simulink model "Mission_Server_LeaderFollower_QBot2_QDrone_Vicon_FrSky"  (Simulink 9.1)
settings: Solver=ode2  StartTime=0.0  StopTime=inf  FixedStep=0.001  RelTol=1e-3  EnableMultiTasking=on
undefined symbols (not defined in the file): Host, localhost, qc_get_step_size
libraries: quarc_library x34, simulink x5
(part 1 of 2)
settings Model: Creator=Admin  LastModifiedBy=jpineros  SimulationMode=external  ExtModeTrigDuration=10000
settings SolverCC: PositivePriorityOrder=on
settings DataIOCC: SaveFormat=Dataset
settings OptimizationCC: LifeSpan=auto
settings DebuggingCC: UnderspecifiedInitializationDetection=Simplified  MergeDetectMultiDrivingBlocksExec=error
settings HardwareCC: ProdBitPerPointer=64  ProdBitPerSizeT=64  ProdBitPerPtrDiffT=64  ProdLargestAtomicFloat=Float  ProdIntDivRoundTo=Zero  ProdEndianess=LittleEndian  ProdWordSize=64  ProdHWDeviceType=Intel->x86-64 (Windows64)
settings ModelReferenceCC: PropagateSignalLabelsOutOfModel=on
settings RTWCC: SystemTargetFile=quarc_win64.tlc  TemplateMakefile=quarc_default_tmf  Description=QUARC Win64 Target  BuildConfiguration=Faster Runs
settings STFCustomTargetCC: ConcurrentExecutionCompliant=on  SystemTargetFile=quarc_win64.tlc
settings GRTTargetCC: TargetPreCompLibLocation=C:\PROGRA~3\QUARC\lib\2018a\win64\release  ParMdlRefBuildCompliant=off  CompOptLevelCompliant=off  MatFileLogging=off  CPPClassGenCompliant=off  UseToolchainInfoCompliant=off  ExtMode=on  ExtModeMexFile=quarc_comm
settings ConfigComp: CovHtmlReporting=off

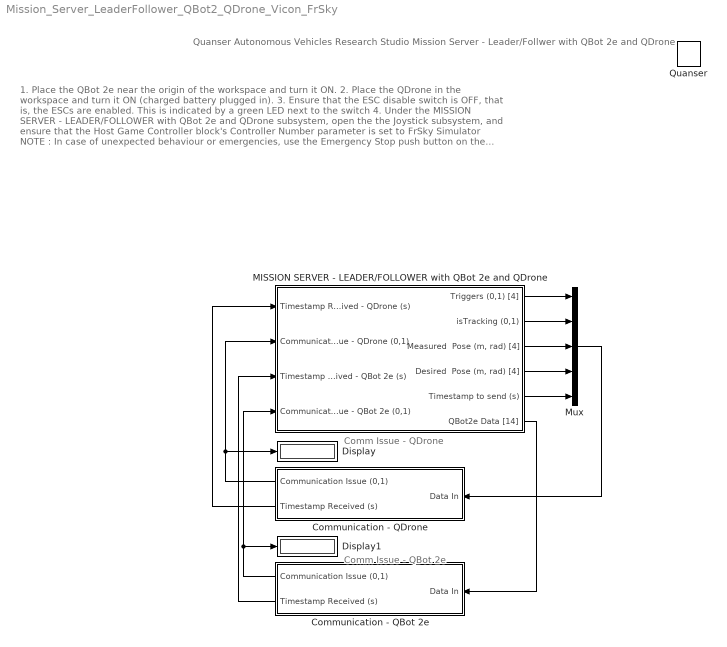
== system Mission_Server_LeaderFollower_QBot2_QDrone_Vicon_FrSky ==
  note: 1. Place the QBot 2e near the origin of the workspace and turn it ON.
      | 2. Place the QDrone in the workspace and turn it ON (charged battery plugged in).
      | 3. Ensure that the ESC disable switch is OFF, that is, the ESCs are enabled. This is indicated by a green LED next to the switch
      | 4. Under the MISSION SERVER - LEADER/FOLLOWER with QBot 2e and QDrone subsystem, open the the Joystick subsystem, and ensure that the Host Game Controller block's Controller Number parameter is set to FrSky Simulator
      | NOTE : In case of unexpected behaviour or emergencies, use the Emergency Stop push button on the Spektrum Joystick to cut all power to the motors (this will result in the drone falling).
      | 5. Open the Data Server (Localization) subsystem and follow the steps there to set up the correct calibration and rigid body definition files for the selected QBot 2e and QDrone.
      | 6. Under the QUARC menu, click on Build .
      | 7. Under the QUARC menu, click on Start . Wait for the model to start running (takes ~1 to 5 seconds for the Motive API to initialize and send localization data).
      | 8. In the MISSION SERVER - LEADER/FOLLOWER with QBot 2e and QDrone subsystem, ensure that the isTracking? display shows 1 and that the Joystick Issue display shows 0 (joystick must be powered ON with USB dongle attached to the PC).
      | 9. Start running the Commander_Stabilizer_QBot2e_Leader.mdl model.
      | 10. Start running the Commander_Stabilizer_QDrone_Follower.mdl model.
      | 11. Arm the drone by moving the Arm/Disarm toggle to the 2 position.
      | 12. Takeoff the drone by moving the Takeoff/Land toggle to the 2 position. The QDrone should takeoff and hover.
      | 13. Toggle the Start/Stop Toggle switch ONCE to start sending waypoint to the Leader (QBot 2e). The QBot 2e should start moving towards the first specified waypoint and the QDrone should follow it.
      | NOTE : The end condition for the FOLLOWER (QDrone) is when the QBot 2e returns to the starting position (when the QDrone model was first started). At that point, the QDrone will be hovering a bit further away (rather than hovering close to/above the QBot 2e) to allow for landing (without hitting the QBot 2e).
      | 14. When finished, move the Takeoff/Land toggle to the 0 position to land the drone. The QDrone should land.
      | 15. Move the Arm/Disarm toggle to the 0 position. (The Commander_Stabilizer_QDrone_Follower.mdl model disarms the drone and stops automatically upon landing).
      | 16. Stop the QBot 2e model. Then stop this model.
  note: Quanser Autonomous Vehicles Research Studio
      | Mission Server - Leader/Follwer with QBot 2e and QDrone
  note: Comm Issue - QDrone
  note: Comm Issue - QBot 2e
  Communication - QBot 2e : Subsystem
  Communication - QDrone : Subsystem
  Display : Display
  Display1 : Display
  MISSION SERVER - LEADER/FOLLOWER with QBot 2e and QDrone : Subsystem
  Mux : Mux  Inputs=5
  Quanser : quarc_library/Logos/Quanser
  wires:
  Communication - QDrone/2(Timestamp Received (s)) -> MISSION SERVER - LEADER/FOLLOWER with QBot 2e and QDrone/1(Timestamp Received - QDrone (s))
  MISSION SERVER - LEADER/FOLLOWER with QBot 2e and QDrone/5(Timestamp to send (s)) -> Mux/5
  Mux/1 -> Communication - QDrone/1(Data In)
  Communication - QDrone/1(Communication Issue (0,1)) -> Display/1, MISSION SERVER - LEADER/FOLLOWER with QBot 2e and QDrone/2(Communication  Issue - QDrone (0,1))
  MISSION SERVER - LEADER/FOLLOWER with QBot 2e and QDrone/3("Measured  Pose (m, rad) [4]") -> Mux/3
  MISSION SERVER - LEADER/FOLLOWER with QBot 2e and QDrone/4("Desired  Pose (m, rad) [4]") -> Mux/4
  Communication - QBot 2e/1(Communication Issue (0,1)) -> MISSION SERVER - LEADER/FOLLOWER with QBot 2e and QDrone/4(Communication  Issue - QBot 2e (0,1)), Display1/1
  Communication - QBot 2e/2(Timestamp Received (s)) -> MISSION SERVER - LEADER/FOLLOWER with QBot 2e and QDrone/3(Timestamp Received - QBot 2e (s))
  MISSION SERVER - LEADER/FOLLOWER with QBot 2e and QDrone/6(QBot2e Data [14]) -> Communication - QBot 2e/1(Data In)
  MISSION SERVER - LEADER/FOLLOWER with QBot 2e and QDrone/1(Triggers (0,1) [4]) -> Mux/1
  MISSION SERVER - LEADER/FOLLOWER with QBot 2e and QDrone/2(isTracking (0,1)) -> Mux/2

== system Mission_Server_LeaderFollower_QBot2_QDrone_Vicon_FrSky/Communication - QBot 2e ==
  note: Argument (-URI_Leader) is set at the MEX-file arguments found at Model Configuration Properties > Code Generation > Interface
      |
      | Format:
      | tcpip://localhost:18001
  Data In : Inport
  Constant : Constant
  Detect Communication loss : Subsystem
  Model Argument : quarc_library/Sources/Signals/Model Argument  argument_name=URI_Leader  has_value=on  data_type_mode=Specify via dialog  data_type=char  max_length=80  default_value=0  variable_size=off
      settings: AttributesFormatString=(-%<argument_name>)  SourceProductName=QUARC Targets
  Stream Server : quarc_library/Communications/Basic/Stream Server  uri_source=External input port  uri=tcpip://localhost:18877  apply_uri_to_all_configs=off  send_buffer_size=1460  receive_buffer_size=1460  byte_order=little endian (Intel - LSB first)  optimization=Minimum latency  send_options=Send most recent data  receive_options=Receive most recent data  default_value=[0]  sample_time=qc_get_step_size  active=off  implementation=Use blocking I/O in a separate thread  send_fifo_size=1000  receive_fifo_size=1000  send_priority=0  receive_priority=0  send_dimensions=off  receive_dimensions=off  max_dimensions=-1  data_type=Inherited via back propagation  type_expr=BusObject
  "String Display " : quarc_library/Strings/String Display  alignment=center  display_mode=Single line  sample_time=-1  use_new=off
      settings: SourceProductName=QUARC Targets
  Terminator1 : Terminator
  Terminator2 : Terminator
  Communication Issue (0,1) : Outport
  Timestamp Received (s) : Outport  Port=2
  wires:
  Data In/1 -> Stream Server/1
  Constant/1 -> Stream Server/2
  Stream Server/3 -> Terminator2/1
  Stream Server/5 -> Terminator1/1
  Model Argument/1 -> "String Display "/1, Stream Server/3
  Stream Server/4 -> Timestamp Received (s)/1
  Stream Server/1 -> Detect Communication loss/1(State)
  Stream Server/2 -> Detect Communication loss/2(Error)
  Detect Communication loss/1(Communication Issue (0,1)) -> Communication Issue (0,1)/1

== system Mission_Server_LeaderFollower_QBot2_QDrone_Vicon_FrSky/Communication - QDrone ==
  note: Argument (-URI_Follower) is set at the MEX-file arguments found at Model Configuration Properties > Code Generation > Interface
      |
      | Format:
      | tcpip://localhost:18002
  Data In : Inport
  Constant : Constant
  Detect Communication loss : Subsystem
  Model Argument : quarc_library/Sources/Signals/Model Argument  argument_name=URI_Follower  has_value=on  data_type_mode=Specify via dialog  data_type=char  max_length=80  default_value=0  variable_size=off
      settings: AttributesFormatString=(-%<argument_name>)  SourceProductName=QUARC Targets
  Stream Server : quarc_library/Communications/Basic/Stream Server  uri_source=External input port  uri=tcpip://localhost:18877  apply_uri_to_all_configs=off  send_buffer_size=1460  receive_buffer_size=1460  byte_order=little endian (Intel - LSB first)  optimization=Minimum latency  send_options=Send most recent data  receive_options=Receive most recent data  default_value=zeros(1,1)  sample_time=qc_get_step_size  active=off  implementation=Use blocking I/O in a separate thread  send_fifo_size=1000  receive_fifo_size=1000  send_priority=0  receive_priority=0  send_dimensions=off  receive_dimensions=off  max_dimensions=-1  data_type=Inherited via back propagation  type_expr=BusObject
  "String Display " : quarc_library/Strings/String Display  alignment=center  display_mode=Single line  sample_time=-1  use_new=off
      settings: SourceProductName=QUARC Targets
  Terminator1 : Terminator
  Terminator2 : Terminator
  Communication Issue (0,1) : Outport
  Timestamp Received (s) : Outport  Port=2
  wires:
  Detect Communication loss/1(Communication Issue (0,1)) -> Communication Issue (0,1)/1
  Stream Server/2 -> Detect Communication loss/2(Error)
  Stream Server/1 -> Detect Communication loss/1(State)
  Stream Server/4 -> Timestamp Received (s)/1
  Model Argument/1 -> Stream Server/3, "String Display "/1
  Stream Server/5 -> Terminator1/1
  Stream Server/3 -> Terminator2/1
  Data In/1 -> Stream Server/1
  Constant/1 -> Stream Server/2

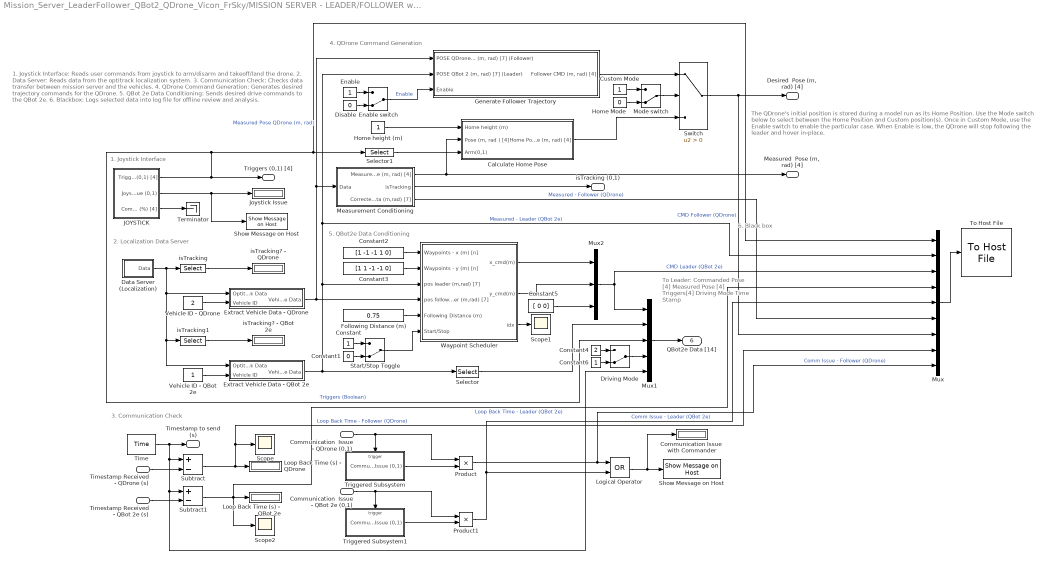
== system Mission_Server_LeaderFollower_QBot2_QDrone_Vicon_FrSky/MISSION SERVER - LEADER/FOLLOWER with QBot 2e and QDrone ==
  note: To Leader:
      | Commanded Pose [4]
      | Measured Pose [4]
      | Triggers[4]
      | Driving Mode
      | Time Stamp
  note: 5. QBot2e Data Conditioning
  note: The QDrone's initial position is stored during a model run as its Home Position.
      | Use the Mode switch below to select between the Home Position and Custom position(s).
      | Once in Custom Mode, use the Enable switch to enable the particular case.
      | When Enable is low, the QDrone will stop following the leader and hover in-place.
  note: 3. Communication Check
  note: 6. Black box
  note: 2. Localization Data Server
  note: 1. Joystick Interface
  note: 4. QDrone Command Generation
  note: 1. Joystick Interface: Reads user commands from joystick to arm/disarm and takeoff/land the drone.
      | 2. Data Server: Reads data from the optitrack localization system.
      | 3. Communication Check: Checks data transfer between mission server and the vehicles.
      | 4. QDrone Command Generation: Generates desired trajectory commands for the QDrone.
      | 5. QBot 2e Data Conditioning: Sends desired drive commands to the QBot 2e.
      | 6. Blackbox: Logs selected data into log file for offline review and analysis.
  Timestamp Received - QDrone (s) : Inport
  Communication  Issue - QDrone (0,1) : Inport  Port=2
  Timestamp Received - QBot 2e (s) : Inport  Port=3
  Communication  Issue - QBot 2e (0,1) : Inport  Port=4
  Calculate Home Pose : Subsystem
  Communication Issue  with Commander : Display
  Constant : Constant
  Constant1 : Constant  Value=0
  Constant2 : Constant  Value=[1 -1 -1 1 0]
  Constant3 : Constant  Value=[1 1 -1 -1 0]
  Constant4 : Constant  Value=2
  Constant5 : Constant  Value=[ 0 0]
  Constant6 : Constant
  Custom Mode : Constant
  "Data Server (Localization) " : Subsystem
  Disable : Constant  Value=0
  Driving Mode : ManualSwitch  CurrentSetting=0
  Enable : Constant
  Enable switch : ManualSwitch  CurrentSetting=0
  Extract Vehicle Data - QBot 2e : Subsystem
  Extract Vehicle Data - QDrone : Subsystem
  Following Distance (m) : Constant  Value=0.75
  Generate Follower Trajectory : Subsystem
  Home Mode : Constant  Value=0
  Home height (m) : Constant
  JOYSTICK : Subsystem
  Joystick Issue : Display
  Logical Operator : Logic  Operator=OR  AllPortsSameDT=off  OutDataTypeStr=boolean
  Loop Back Time (s) - QBot 2e : Display
  Loop Back Time (s) - QDrone : Display
  Measurement Conditioning : Subsystem
  Mode switch : ManualSwitch  CurrentSetting=0
  Mux : Mux  Inputs=9
  Mux1 : Mux  Inputs=5
  Mux2 : Mux  Inputs=3
  Product : Product
  Product1 : Product
  Scope : Scope
  Scope1 : Scope
  Scope2 : Scope
  Selector : Selector  InputPortWidth=7  IndexOptions=Index vector (dialog)  Indices=[1:3 6]  OutputSizes=1
  Selector1 : Selector  InputPortWidth=4  IndexOptions=Index vector (dialog)  Indices=[1]  OutputSizes=1
  Show Message on Host : quarc_library/Sinks/Error Handling/Show Message on Host  message_type=Fixed error message  message_icon=Warning  message=Mission Server: Communication Issue with QDrone or QBot 2e
      settings: AttributesFormatString="\"%<message>\""  SourceProductName=QUARC Targets
  "Show Message on Host " : quarc_library/Sinks/Error Handling/Show Message on Host  message_type=Fixed error message  message_icon=Warning  message=Mission Server: Joystick Disconnected
      settings: AttributesFormatString="\"%<message>\""  SourceProductName=QUARC Targets
  Start/Stop Toggle : ManualSwitch  CurrentSetting=0
  Subtract : Sum  Inputs=+-
  Subtract1 : Sum  Inputs=+-
  Switch : Switch  Criteria=u2 > Threshold
  Terminator : Terminator
  Time : quarc_library/Sources/Time/Time  time_source=Wall clock  sample_time=qc_get_step_size
  To Host File : quarc_library/Sinks/To Host/To Host File  file_name=saved_data/%m/Mission_Server_%{date}_%{time}.mat  variable_name=mission_server_data  decimation=1  sample_time=-1  file_format=MAT-file v.5  options=No header or footer  append=off  final_file_name=saved_data/Mission_Server_LeaderFollower_QBot2_QDrone_Vicon_FrSky/Mission_Server_20-Jan-2022_08-52-01.mat  bitrate=2000000
  Triggered Subsystem : Subsystem  TreatAsAtomicUnit=on
  Triggered Subsystem1 : Subsystem  TreatAsAtomicUnit=on
  Vehicle ID - QBot 2e : Constant
  Vehicle ID - QDrone : Constant  Value=2
  Waypoint Scheduler : Subsystem
  isTracking : Selector  InputPortWidth=14  IndexOptions=Index vector (dialog)  Indices=[13]  OutputSizes=1
  isTracking1 : Selector  InputPortWidth=14  IndexOptions=Index vector (dialog)  Indices=[14]  OutputSizes=1
  isTracking? - QBot 2e : Display
  isTracking? - QDrone : Display
  Triggers (0,1) [4] : Outport
  isTracking (0,1) : Outport  Port=2
  "Measured  Pose (m, rad) [4]" : Outport  Port=3
  "Desired  Pose (m, rad) [4]" : Outport  Port=4
  Timestamp to send (s) : Outport  Port=5
  QBot2e Data [14] : Outport  Port=6
  wires:
  Communication  Issue - QDrone (0,1)/1 -> Product/1, Triggered Subsystem/Trigger
  isTracking/1 -> isTracking? - QDrone/1
  JOYSTICK/2(Joystick Issue (0,1)) -> Joystick Issue/1, "Show Message on Host "/1
  JOYSTICK/3(Commands (%) [4]) -> Terminator/1
  Time/1 -> Mux1/5, Subtract1/1, Subtract/1, Timestamp to send (s)/1
  Timestamp Received - QDrone (s)/1 -> Subtract/2
  Subtract/1 -> Loop Back Time (s) - QDrone/1, Scope/1, Mux/8  "Loop Back Time - Follower (QDrone)"
  Switch/1 -> Mux/7, "Desired  Pose (m, rad) [4]"/1  "CMD Follower (QDrone)"
  Measurement Conditioning/2(isTracking) -> isTracking (0,1)/1
  Measurement Conditioning/1("Measured Pose (m, rad) [4]") -> "Measured  Pose (m, rad) [4]"/1, Calculate Home Pose/2("Pose (m, rad ) [4]")
  "Data Server (Localization) "/1(Data) -> Extract Vehicle Data - QDrone/1(Optitrack Data), Extract Vehicle Data - QBot 2e/1(Optitrack Data), isTracking1/1, isTracking/1
  Vehicle ID - QDrone/1 -> Extract Vehicle Data - QDrone/2(Vehicle ID)
  Calculate Home Pose/1("Home Pose (m, rad) [4]") -> Switch/3
  Home height (m)/1 -> Calculate Home Pose/1(Home height (m))
  Triggered Subsystem/1(Communication Issue (0,1)) -> Product/2
  Product/1 -> Logical Operator/1, Mux/9  "Comm Issue - Follower (QDrone)"
  Mux/1 -> To Host File/1
  Custom Mode/1 -> Mode switch/1
  Mode switch/1 -> Switch/2
  Home Mode/1 -> Mode switch/2
  Enable/1 -> Enable switch/1
  Disable/1 -> Enable switch/2
  Enable switch/1 -> Generate Follower Trajectory/3(Enable)  "Enable"
  Generate Follower Trajectory/1("Follower CMD (m, rad) [4]") -> Switch/1
  Vehicle ID - QBot 2e/1 -> Extract Vehicle Data - QBot 2e/2(Vehicle ID)
  Timestamp Received - QBot 2e (s)/1 -> Subtract1/2
  Subtract1/1 -> Scope2/1, Loop Back Time (s) - QBot 2e/1, Mux/4  "Loop Back Time - Leader (QBot 2e)"
  Logical Operator/1 -> Show Message on Host/1, Communication Issue  with Commander/1
  Product1/1 -> Logical Operator/2, Mux/5  "Comm Issue - Leader (QBot 2e)"
  Triggered Subsystem1/1(Communication Issue (0,1)) -> Product1/2
  Communication  Issue - QBot 2e (0,1)/1 -> Triggered Subsystem1/Trigger, Product1/1
  Following Distance (m)/1 -> Waypoint Scheduler/5(Following Distance (m))
  Constant2/1 -> Waypoint Scheduler/1(Waypoints - x (m) [n])
  Constant3/1 -> Waypoint Scheduler/2(Waypoints - y (m) [n])
  Constant/1 -> Start/Stop Toggle/1
  Constant1/1 -> Start/Stop Toggle/2
  Extract Vehicle Data - QBot 2e/1(Vehicle Data) -> Generate Follower Trajectory/2("POSE QBot 2 (m, rad) [7] (Leader)"), Mux/2, Waypoint Scheduler/3(pos leader (m,rad) [7]), Selector/1  "Measured - Leader (QBot 2e)"
  Extract Vehicle Data - QDrone/1(Vehicle Data) -> Waypoint Scheduler/4(pos follower (m,rad) [7]), Measurement Conditioning/1(Data), Generate Follower Trajectory/1("POSE QDrone (m, rad) [7] (Follower)")  "Measured Pose QDrone (m, rad)"
  isTracking1/1 -> isTracking? - QBot 2e/1
  Constant5/1 -> Mux2/3
  Mux2/1 -> Mux/3, Mux1/1  "CMD Leader (QBot 2e)"
  JOYSTICK/1(Triggers (0,1) [4]) -> Triggers (0,1) [4]/1, Mux/1, Selector1/1, Mux1/3  "Triggers (Boolean)"
  Driving Mode/1 -> Mux1/4
  Constant4/1 -> Driving Mode/1
  Constant6/1 -> Driving Mode/2
  Mux1/1 -> QBot2e Data [14]/1
  Waypoint Scheduler/2(y_cmd(m)) -> Mux2/2
  Waypoint Scheduler/1(x_cmd(m)) -> Mux2/1
  Waypoint Scheduler/3(idx) -> Scope1/1
  Start/Stop Toggle/1 -> Waypoint Scheduler/6(Start/Stop)
  Selector/1 -> Mux1/2
  Selector1/1 -> Calculate Home Pose/3(Arm(0,1))
  Measurement Conditioning/3(Corrected Pose Data (m,rad) [7]) -> Mux/6  "Measured - Follower (QDrone)"

== system Mission_Server_LeaderFollower_QBot2_QDrone_Vicon_FrSky/Communication - QBot 2e/Detect Communication loss ==
  note: Check if stream is 2 (connected) and error is positive (error codes are negative). Otherwise issue a communication error.
  State : Inport
  Error : Inport  Port=2
  Data Type Conversion : DataTypeConversion
  MATLAB Function : MATLAB Function  TreatAsAtomicUnit=on
  Terminator2 : Terminator
  Threshold : quarc_library/Discontinuities/Threshold  operator=>=  param_src=Specify via dialog  threshold=0.5  duration=0.1
      settings: SourceProductName=QUARC Targets
  Time : quarc_library/Sources/Time/Time  time_source=Wall clock  sample_time=qc_get_step_size
  Communication Issue (0,1) : Outport
  wires:
  Error/1 -> MATLAB Function/3(error)
  MATLAB Function/1(stream_connection_loss) -> Threshold/1
  State/1 -> MATLAB Function/2(state)
  Time/1 -> MATLAB Function/1(time)
  Threshold/2 -> Terminator2/1
  Data Type Conversion/1 -> Communication Issue (0,1)/1
  Threshold/1 -> Data Type Conversion/1

== system Mission_Server_LeaderFollower_QBot2_QDrone_Vicon_FrSky/Communication - QDrone/Detect Communication loss ==
  note: Check if stream is 2 (connected) and error is positive (error codes are negative). Otherwise issue a communication error.
  State : Inport
  Error : Inport  Port=2
  Data Type Conversion : DataTypeConversion
  MATLAB Function : MATLAB Function  TreatAsAtomicUnit=on
  Terminator2 : Terminator
  Threshold : quarc_library/Discontinuities/Threshold  operator=>=  param_src=Specify via dialog  threshold=0.5  duration=0.1
      settings: SourceProductName=QUARC Targets
  Time : quarc_library/Sources/Time/Time  time_source=Wall clock  sample_time=qc_get_step_size
  Communication Issue (0,1) : Outport
  wires:
  Threshold/1 -> Data Type Conversion/1
  Data Type Conversion/1 -> Communication Issue (0,1)/1
  Threshold/2 -> Terminator2/1
  Time/1 -> MATLAB Function/1(time)
  State/1 -> MATLAB Function/2(state)
  MATLAB Function/1(stream_connection_loss) -> Threshold/1
  Error/1 -> MATLAB Function/3(error)

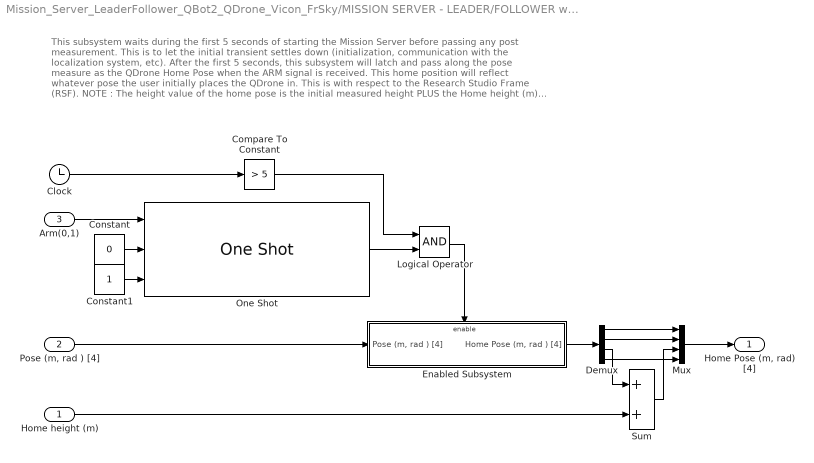
== system Mission_Server_LeaderFollower_QBot2_QDrone_Vicon_FrSky/MISSION SERVER - LEADER/FOLLOWER with QBot 2e and QDrone/Calculate Home Pose ==
  note: This subsystem waits during the first 5 seconds of starting the Mission Server before passing any post measurement.
      | This is to let the initial transient settles down (initialization, communication with the localization system, etc).
      | After the first 5 seconds, this subsystem will latch and pass along the pose measure as the QDrone Home Pose when
      | the ARM signal is received.
      | This home position will reflect whatever pose the user initially places the QDrone in.
      | This is with respect to the Research Studio Frame (RSF).
      |
      | NOTE : The height value of the home pose is the initial measured height PLUS the Home height (m) input value.
  Home height (m) : Inport
  "Pose (m, rad ) [4]" : Inport  Port=2
  Arm(0,1) : Inport  Port=3
  Clock : Clock
  Compare To Constant : simulink/Logic and Bit Operations/Compare To Constant  relop=>  const=5  OutDataTypeStr=boolean
  Constant : Constant  Value=0
  Constant1 : Constant
  Demux : Demux
  Enabled Subsystem : Subsystem  TreatAsAtomicUnit=on
  Logical Operator : Logic  AllPortsSameDT=off  OutDataTypeStr=boolean
  Mux : Mux
  One Shot : quarc_library/Discontinuities/One Shot  trigger_type=Rising edge  redun_pulse=Ignore extraneous pulse  width_source=Specify via dialog  pulse_width=1/qc_get_step_size
      settings: SourceProductName=QUARC Targets
  Sum : Sum
  "Home Pose (m, rad) [4]" : Outport
  wires:
  Constant/1 -> One Shot/2
  Constant1/1 -> One Shot/3
  Arm(0,1)/1 -> One Shot/1
  One Shot/1 -> Logical Operator/2
  "Pose (m, rad ) [4]"/1 -> Enabled Subsystem/1("Pose (m, rad ) [4] ")
  Clock/1 -> Compare To Constant/1
  Compare To Constant/1 -> Logical Operator/1
  Logical Operator/1 -> Enabled Subsystem/Enable
  Enabled Subsystem/1("Home Pose (m, rad ) [4]") -> Demux/1
  Demux/1 -> Mux/1
  Demux/2 -> Mux/2
  Demux/4 -> Mux/4
  Demux/3 -> Sum/1
  Sum/1 -> Mux/3
  Home height (m)/1 -> Sum/2
  Mux/1 -> "Home Pose (m, rad) [4]"/1

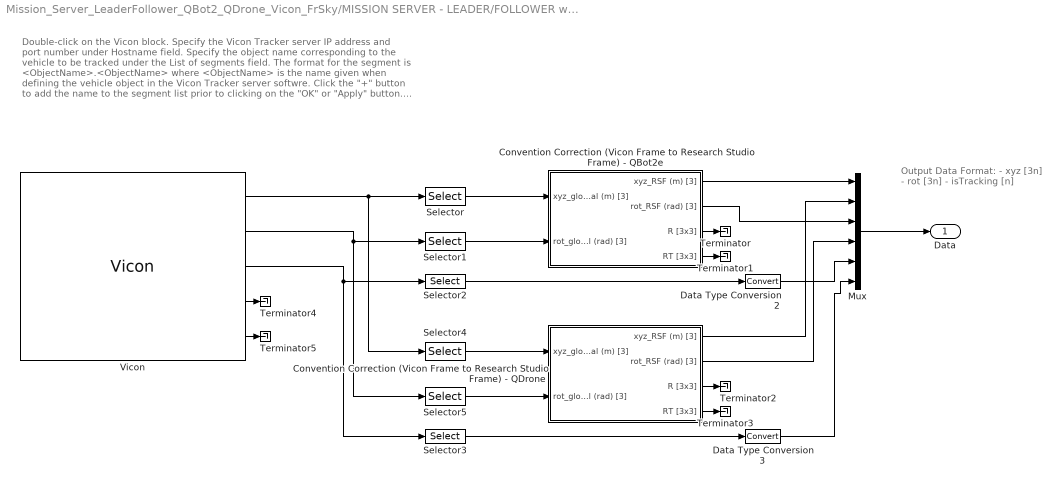
== system Mission_Server_LeaderFollower_QBot2_QDrone_Vicon_FrSky/MISSION SERVER - LEADER/FOLLOWER with QBot 2e and QDrone/Data Server (Localization)  ==
  note: Output Data Format:
      | - xyz [3n]
      | - rot [3n]
      | - isTracking [n]
  note: Double-click on the Vicon block.
      |
      | Specify the Vicon Tracker server IP address and port number under Hostname field.
      |
      | Specify the object name corresponding to the vehicle to be tracked under the
      | List of segments field. The format for the segment is <ObjectName>.<ObjectName>
      | where <ObjectName> is the name given when defining the vehicle object in the
      | Vicon Tracker server softwre. Click the "+" button to add the name to the segment list
      | prior to clicking on the "OK" or "Apply" button.
      | Remove extra/unused entries from the list using the "-" button.
  Convention Correction (Vicon Frame to Research Studio Frame) - QBot2e : Subsystem
  Convention Correction (Vicon Frame to Research Studio Frame) - QDrone : Subsystem
  Data Type Conversion2 : DataTypeConversion
  Data Type Conversion3 : DataTypeConversion
  Mux : Mux  Inputs=6
  Selector : Selector  InputPortWidth=6  IndexOptions=Index vector (dialog)  Indices=[1:3]  OutputSizes=1
  Selector1 : Selector  InputPortWidth=6  IndexOptions=Index vector (dialog)  Indices=[1:3]  OutputSizes=1
  Selector2 : Selector  InputPortWidth=2  IndexOptions=Index vector (dialog)  Indices=[1]  OutputSizes=1
  Selector3 : Selector  InputPortWidth=2  IndexOptions=Index vector (dialog)  Indices=[2]  OutputSizes=1
  Selector4 : Selector  InputPortWidth=6  IndexOptions=Index vector (dialog)  Indices=[4:6]  OutputSizes=1
  Selector5 : Selector  InputPortWidth=6  IndexOptions=Index vector (dialog)  Indices=[4:6]  OutputSizes=1
  Terminator{,1..5} (6 alike) : Terminator
  Vicon : quarc_library/Devices/Third-Party/Vicon/Vicon  hostname=localhost:801  segment_list=ObjectName.ObjectName\0ObjectName.ObjectName\0\0  marker_list=\0  unlabeled_markers=[]  stream_mode=2  sample_time=qc_get_step_size  num_segments=2  num_markers=0  active=on
      settings: SourceProductName=QUARC Targets
  Data : Outport
  wires:
  Convention Correction (Vicon Frame to Research Studio Frame) - QDrone/4(RT [3x3]) -> Terminator3/1
  Convention Correction (Vicon Frame to Research Studio Frame) - QDrone/3(R [3x3]) -> Terminator2/1
  Convention Correction (Vicon Frame to Research Studio Frame) - QBot2e/4(RT [3x3]) -> Terminator1/1
  Convention Correction (Vicon Frame to Research Studio Frame) - QBot2e/3(R [3x3]) -> Terminator/1
  Vicon/5 -> Terminator5/1
  Vicon/4 -> Terminator4/1
  Convention Correction (Vicon Frame to Research Studio Frame) - QDrone/2(rot_RSF (rad) [3]) -> Mux/4
  Convention Correction (Vicon Frame to Research Studio Frame) - QBot2e/2(rot_RSF (rad) [3]) -> Mux/3
  Mux/1 -> Data/1
  Selector5/1 -> Convention Correction (Vicon Frame to Research Studio Frame) - QDrone/2(rot_global (rad) [3])
  Selector4/1 -> Convention Correction (Vicon Frame to Research Studio Frame) - QDrone/1(xyz_global (m) [3])
  Selector/1 -> Convention Correction (Vicon Frame to Research Studio Frame) - QBot2e/1(xyz_global (m) [3])
  Vicon/1 -> Selector/1, Selector4/1
  Selector3/1 -> Data Type Conversion3/1
  Selector2/1 -> Data Type Conversion2/1
  Selector1/1 -> Convention Correction (Vicon Frame to Research Studio Frame) - QBot2e/2(rot_global (rad) [3])
  Vicon/2 -> Selector1/1, Selector5/1
  Convention Correction (Vicon Frame to Research Studio Frame) - QDrone/1(xyz_RSF (m) [3]) -> Mux/2
  Vicon/3 -> Selector2/1, Selector3/1
  Data Type Conversion3/1 -> Mux/6
  Data Type Conversion2/1 -> Mux/5
  Convention Correction (Vicon Frame to Research Studio Frame) - QBot2e/1(xyz_RSF (m) [3]) -> Mux/1

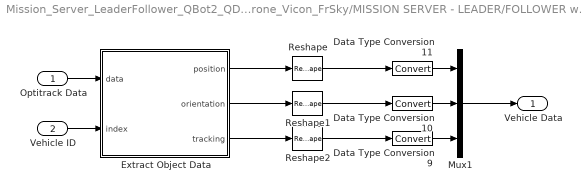
== system Mission_Server_LeaderFollower_QBot2_QDrone_Vicon_FrSky/MISSION SERVER - LEADER/FOLLOWER with QBot 2e and QDrone/Extract Vehicle Data - QBot 2e ==
  Optitrack Data : Inport
  Vehicle ID : Inport  Port=2
  Data Type Conversion10 : DataTypeConversion
  Data Type Conversion11 : DataTypeConversion
  Data Type Conversion9 : DataTypeConversion
  Extract Object Data : MATLAB Function  TreatAsAtomicUnit=on
  Mux1 : Mux  Inputs=3
  Reshape : Reshape
  Reshape1 : Reshape
  Reshape2 : Reshape
  Vehicle Data : Outport
  wires:
  Reshape2/1 -> Data Type Conversion9/1
  Reshape1/1 -> Data Type Conversion10/1
  Reshape/1 -> Data Type Conversion11/1
  Data Type Conversion9/1 -> Mux1/3
  Data Type Conversion10/1 -> Mux1/2
  Data Type Conversion11/1 -> Mux1/1
  Extract Object Data/2(orientation) -> Reshape1/1
  Extract Object Data/3(tracking) -> Reshape2/1
  Extract Object Data/1(position) -> Reshape/1
  Mux1/1 -> Vehicle Data/1
  Optitrack Data/1 -> Extract Object Data/1(data)
  Vehicle ID/1 -> Extract Object Data/2(index)

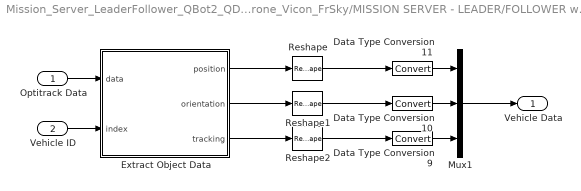
== system Mission_Server_LeaderFollower_QBot2_QDrone_Vicon_FrSky/MISSION SERVER - LEADER/FOLLOWER with QBot 2e and QDrone/Extract Vehicle Data - QDrone ==
  Optitrack Data : Inport
  Vehicle ID : Inport  Port=2
  Data Type Conversion10 : DataTypeConversion
  Data Type Conversion11 : DataTypeConversion
  Data Type Conversion9 : DataTypeConversion
  Extract Object Data : MATLAB Function  TreatAsAtomicUnit=on
  Mux1 : Mux  Inputs=3
  Reshape : Reshape
  Reshape1 : Reshape
  Reshape2 : Reshape
  Vehicle Data : Outport
  wires:
  Reshape2/1 -> Data Type Conversion9/1
  Reshape1/1 -> Data Type Conversion10/1
  Reshape/1 -> Data Type Conversion11/1
  Data Type Conversion9/1 -> Mux1/3
  Data Type Conversion10/1 -> Mux1/2
  Data Type Conversion11/1 -> Mux1/1
  Extract Object Data/2(orientation) -> Reshape1/1
  Extract Object Data/3(tracking) -> Reshape2/1
  Extract Object Data/1(position) -> Reshape/1
  Mux1/1 -> Vehicle Data/1
  Optitrack Data/1 -> Extract Object Data/1(data)
  Vehicle ID/1 -> Extract Object Data/2(index)

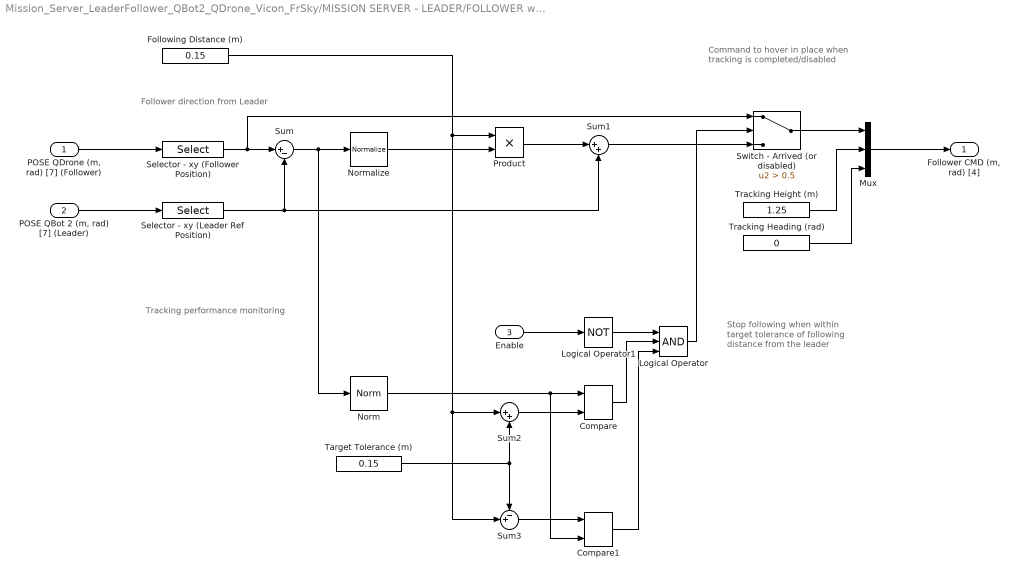
== system Mission_Server_LeaderFollower_QBot2_QDrone_Vicon_FrSky/MISSION SERVER - LEADER/FOLLOWER with QBot 2e and QDrone/Generate Follower Trajectory ==
  note: Command to hover in place when
      | tracking is completed/disabled
  note: Stop following when
      | within target tolerance
      | of following distance from
      | the leader
  note: Tracking performance monitoring
  note: Follower direction from Leader
  "POSE QDrone (m, rad) [7] (Follower)" : Inport
  "POSE QBot 2 (m, rad) [7] (Leader)" : Inport  Port=2
  Enable : Inport  Port=3
  Compare : quarc_library/Logic Operations/Compare  operator=<=  output_data_type=boolean
      settings: SourceProductName=QUARC Targets
  Compare1 : quarc_library/Logic Operations/Compare  operator=>=  output_data_type=boolean
      settings: SourceProductName=QUARC Targets
  Following Distance (m) : Constant  Value=0.15
  Logical Operator : Logic  Inputs=3  AllPortsSameDT=off  OutDataTypeStr=boolean
  Logical Operator1 : Logic  Operator=NOT  Inputs=1  AllPortsSameDT=off  OutDataTypeStr=boolean
  Mux : Mux  Inputs=3
  Norm : quarc_library/Math Operations/Vectors/Norm
      settings: SourceProductName=QUARC Targets
  Normalize : quarc_library/Math Operations/Vectors/Normalize
      settings: SourceProductName=QUARC Targets
  Product : Product
  Selector - xy (Follower Position) : Selector  InputPortWidth=7  IndexOptions=Index vector (dialog)  Indices=[1 2]  OutputSizes=1
  Selector - xy (Leader Ref Position) : Selector  InputPortWidth=7  IndexOptions=Index vector (dialog)  Indices=[1 2]  OutputSizes=1
  Sum : Sum  Inputs=|+-
  Sum1 : Sum  Inputs=|++
  Sum2 : Sum  Inputs=|++
  Sum3 : Sum  Inputs=-+|
  Switch - Arrived (or disabled) : Switch  Criteria=u2 > Threshold  Threshold=0.5
  Target Tolerance (m) : Constant  Value=0.15
  Tracking Heading (rad) : Constant  Value=0
  Tracking Height (m) : Constant  Value=1.25
  "Follower CMD (m, rad) [4]" : Outport
  wires:
  "POSE QDrone (m, rad) [7] (Follower)"/1 -> Selector - xy (Follower Position)/1
  "POSE QBot 2 (m, rad) [7] (Leader)"/1 -> Selector - xy (Leader Ref Position)/1
  Selector - xy (Follower Position)/1 -> Switch - Arrived (or disabled)/1, Sum/1
  Selector - xy (Leader Ref Position)/1 -> Sum1/2, Sum/2
  Sum/1 -> Norm/1, Normalize/1
  Product/1 -> Sum1/1
  Normalize/1 -> Product/2
  Following Distance (m)/1 -> Product/1, Sum2/1, Sum3/2
  Tracking Height (m)/1 -> Mux/2
  Tracking Heading (rad)/1 -> Mux/3
  Sum1/1 -> Switch - Arrived (or disabled)/3
  Switch - Arrived (or disabled)/1 -> Mux/1
  Mux/1 -> "Follower CMD (m, rad) [4]"/1
  Sum2/1 -> Compare/2
  Sum3/1 -> Compare1/1
  Target Tolerance (m)/1 -> Sum2/2, Sum3/1
  Norm/1 -> Compare1/2, Compare/1
  Enable/1 -> Logical Operator1/1
  Logical Operator1/1 -> Logical Operator/1
  Compare/1 -> Logical Operator/2
  Compare1/1 -> Logical Operator/3
  Logical Operator/1 -> Switch - Arrived (or disabled)/2

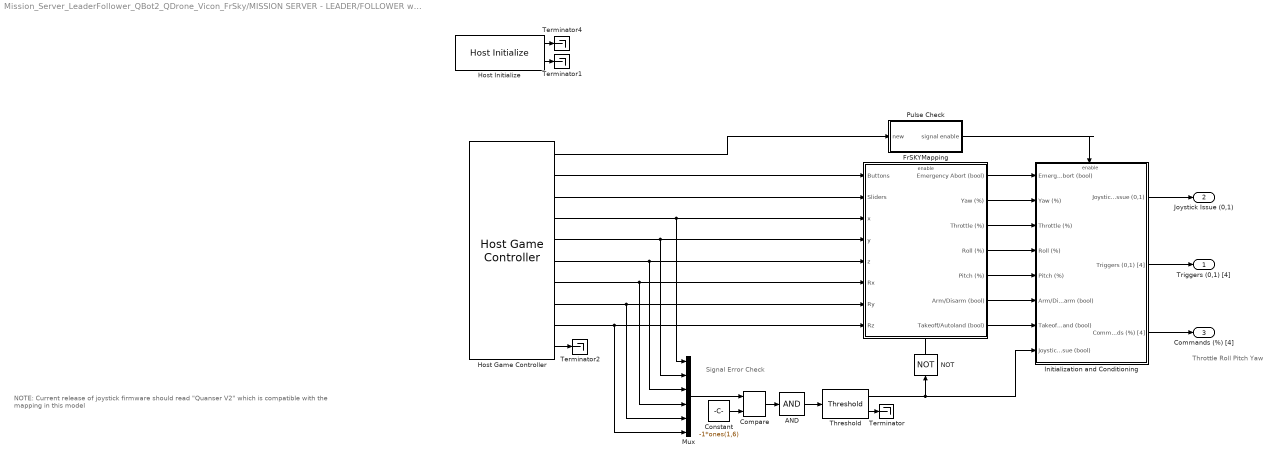
== system Mission_Server_LeaderFollower_QBot2_QDrone_Vicon_FrSky/MISSION SERVER - LEADER/FOLLOWER with QBot 2e and QDrone/JOYSTICK ==
  note: Throttle
      | Roll
      | Pitch
      | Yaw
  note: Signal Error Check
  note: NOTE: Current release of joystick firmware should read "Quanser V2" which is compatible with the mapping in this model
  AND : Logic  Inputs=1  AllPortsSameDT=off  OutDataTypeStr=boolean
  Compare : quarc_library/Logic Operations/Compare  operator===  output_data_type=boolean
      settings: SourceProductName=QUARC Targets
  Constant : Constant  Value=-1*ones(1,6)
  FrSKYMapping : Subsystem
  Host Game Controller : quarc_library/Devices/Peripherals/Host/Host Game Controller  object_name=Host-1  controller=1  buffer_size=20  deadzone=[]  saturation=[]  sample_time=qc_get_step_size  auto_center=off  enabled=on  debug_mode=off
      settings: SourceProductName=QUARC Targets
  Host Initialize : quarc_library/Devices/Peripherals/Host/Host Initialize  object_name=Host-1  uri_source=Use external mode communications  uri=tcpip://localhost:18001  apply_uri_to_all_configs=on  send_buffer_size=1000  receive_buffer_size=1000  thread_priority=0  run_client=on  use_window=off  window_position=[]  sample_time=qc_get_step_size  active=on
      settings: SourceProductName=QUARC Targets
  Initialization and Conditioning : Subsystem  TreatAsAtomicUnit=on
  Mux : Mux  Inputs=6
  NOT : Logic  Operator=NOT  IconShape=distinctive  AllPortsSameDT=off  OutDataTypeStr=boolean
  Pulse Check : Subsystem  TreatAsAtomicUnit=on
  Terminator{,1..2,4} (4 alike) : Terminator
  Threshold : quarc_library/Discontinuities/Threshold  operator=>=  param_src=Specify via dialog  threshold=0.5  duration=0.2
      settings: SourceProductName=QUARC Targets
  Triggers (0,1) [4] : Outport
  Joystick Issue (0,1) : Outport  Port=2
  Commands (%) [4] : Outport  Port=3
  wires:
  Initialization and Conditioning/1(Joystick Issue (0,1)) -> Joystick Issue (0,1)/1
  Host Game Controller/10 -> Terminator2/1
  Host Initialize/1 -> Terminator4/1
  Host Initialize/2 -> Terminator1/1
  Initialization and Conditioning/2(Triggers (0,1) [4]) -> Triggers (0,1) [4]/1
  Initialization and Conditioning/3(Commands (%) [4]) -> Commands (%) [4]/1
  AND/1 -> Threshold/1
  NOT/1 -> FrSKYMapping/Enable
  Threshold/1 -> Initialization and Conditioning/8(Joystick Issue (bool)), NOT/1
  Host Game Controller/3 -> FrSKYMapping/2(Sliders)
  Host Game Controller/2 -> FrSKYMapping/1(Buttons)
  Threshold/2 -> Terminator/1
  Compare/1 -> AND/1
  Constant/1 -> Compare/2
  Mux/1 -> Compare/1
  Host Game Controller/9 -> FrSKYMapping/8(Rz), Mux/6
  Host Game Controller/8 -> FrSKYMapping/7(Ry), Mux/5
  Host Game Controller/7 -> FrSKYMapping/6(Rx), Mux/4
  Host Game Controller/6 -> FrSKYMapping/5(z), Mux/3
  Host Game Controller/5 -> FrSKYMapping/4(y), Mux/2
  Host Game Controller/4 -> FrSKYMapping/3(x), Mux/1
  FrSKYMapping/7(Takeoff/Autoland (bool)) -> Initialization and Conditioning/7(Takeoff/AutoLand (bool))
  Pulse Check/1(signal enable) -> Initialization and Conditioning/Enable
  Host Game Controller/1 -> Pulse Check/1(new)
  FrSKYMapping/4(Roll (%)) -> Initialization and Conditioning/4(Roll (%))
  FrSKYMapping/6("Arm/Disarm (bool) ") -> Initialization and Conditioning/6(Arm/Disarm (bool))
  FrSKYMapping/5(Pitch (%)) -> Initialization and Conditioning/5(Pitch (%))
  FrSKYMapping/1(Emergency Abort (bool)) -> Initialization and Conditioning/1(Emergency Abort (bool))
  FrSKYMapping/3(Throttle (%)) -> Initialization and Conditioning/3(Throttle (%))
  FrSKYMapping/2(Yaw (%)) -> Initialization and Conditioning/2(Yaw (%))

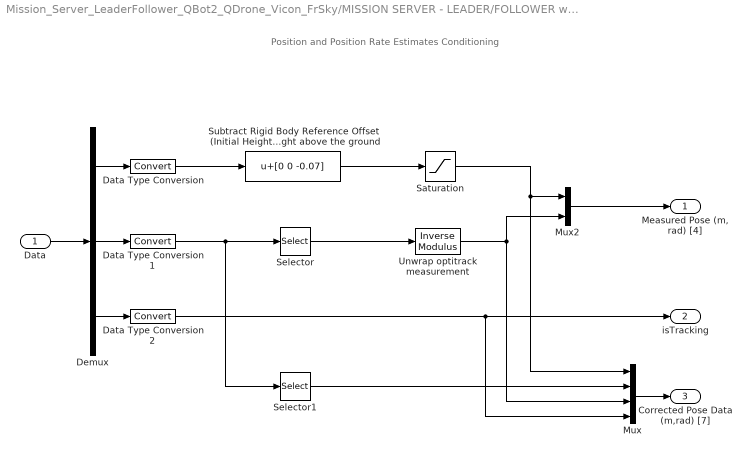
== system Mission_Server_LeaderFollower_QBot2_QDrone_Vicon_FrSky/MISSION SERVER - LEADER/FOLLOWER with QBot 2e and QDrone/Measurement Conditioning ==
  note: Position and Position Rate Estimates Conditioning
  Data : Inport
  Data Type Conversion : DataTypeConversion
  Data Type Conversion1 : DataTypeConversion
  Data Type Conversion2 : DataTypeConversion
  Demux : Demux  Outputs=[3 3 1]
  Mux : Mux
  Mux2 : Mux  Inputs=[3 1]
  Saturation : Saturate  UpperLimit=[2 2 5]  LowerLimit=[-2 -2 0]
  Selector : Selector  InputPortWidth=3  IndexOptions=Index vector (dialog)  Indices=[3]  OutputSizes=1
  Selector1 : Selector  InputPortWidth=3  IndexOptions=Index vector (dialog)  Indices=[1,2]  OutputSizes=1
  Subtract Rigid Body Reference Offset  (Initial Height)  to get height above the ground : Bias  Bias=[0 0 -0.07]
  Unwrap optitrack measurement : quarc_library/Discontinuities/Inverse Modulus  modulus=2*pi  output_derivative=off  output_revolutions=off  max_x=Inf  min_x=-Inf
  "Measured Pose (m, rad) [4]" : Outport
  isTracking : Outport  Port=2
  Corrected Pose Data (m,rad) [7] : Outport  Port=3
  wires:
  Demux/2 -> Data Type Conversion1/1
  Demux/1 -> Data Type Conversion/1
  Demux/3 -> Data Type Conversion2/1
  Mux2/1 -> "Measured Pose (m, rad) [4]"/1
  Data/1 -> Demux/1
  Data Type Conversion2/1 -> Mux/4, isTracking/1
  Subtract Rigid Body Reference Offset  (Initial Height)  to get height above the ground/1 -> Saturation/1
  Saturation/1 -> Mux2/1, Mux/1
  Data Type Conversion1/1 -> Selector1/1, Selector/1
  Selector/1 -> Unwrap optitrack measurement/1
  Data Type Conversion/1 -> Subtract Rigid Body Reference Offset  (Initial Height)  to get height above the ground/1
  Unwrap optitrack measurement/1 -> Mux/3, Mux2/2
  Mux/1 -> Corrected Pose Data (m,rad) [7]/1
  Selector1/1 -> Mux/2

== system Mission_Server_LeaderFollower_QBot2_QDrone_Vicon_FrSky/MISSION SERVER - LEADER/FOLLOWER with QBot 2e and QDrone/Triggered Subsystem ==
  note: This looks for the first falling edge of the communication issue before allowing a communication issue to be triggered,
      | because the mission server model starts first.
  Trigger : TriggerPort  TriggerType=falling  VariantControl=Variant
  Add : Sum
  Compare To Constant : simulink/Logic and Bit Operations/Compare To Constant  relop=>=  const=1  OutDataTypeStr=boolean
  Constant : Constant
  Memory : Memory  InheritSampleTime=on
  Communication Issue (0,1) : Outport  InitialOutput=0
  wires:
  Constant/1 -> Add/1
  Memory/1 -> Add/2
  Add/1 -> Compare To Constant/1, Memory/1
  Compare To Constant/1 -> Communication Issue (0,1)/1

== system Mission_Server_LeaderFollower_QBot2_QDrone_Vicon_FrSky/MISSION SERVER - LEADER/FOLLOWER with QBot 2e and QDrone/Triggered Subsystem1 ==
  note: This looks for the first falling edge of the communication issue before allowing a communication issue to be triggered,
      | because the mission server model starts first.
  Trigger : TriggerPort  TriggerType=falling  VariantControl=Variant
  Add : Sum
  Compare To Constant : simulink/Logic and Bit Operations/Compare To Constant  relop=>=  const=1  OutDataTypeStr=boolean
  Constant : Constant
  Memory : Memory  InheritSampleTime=on
  Communication Issue (0,1) : Outport  InitialOutput=0
  wires:
  Compare To Constant/1 -> Communication Issue (0,1)/1
  Add/1 -> Memory/1, Compare To Constant/1
  Memory/1 -> Add/2
  Constant/1 -> Add/1

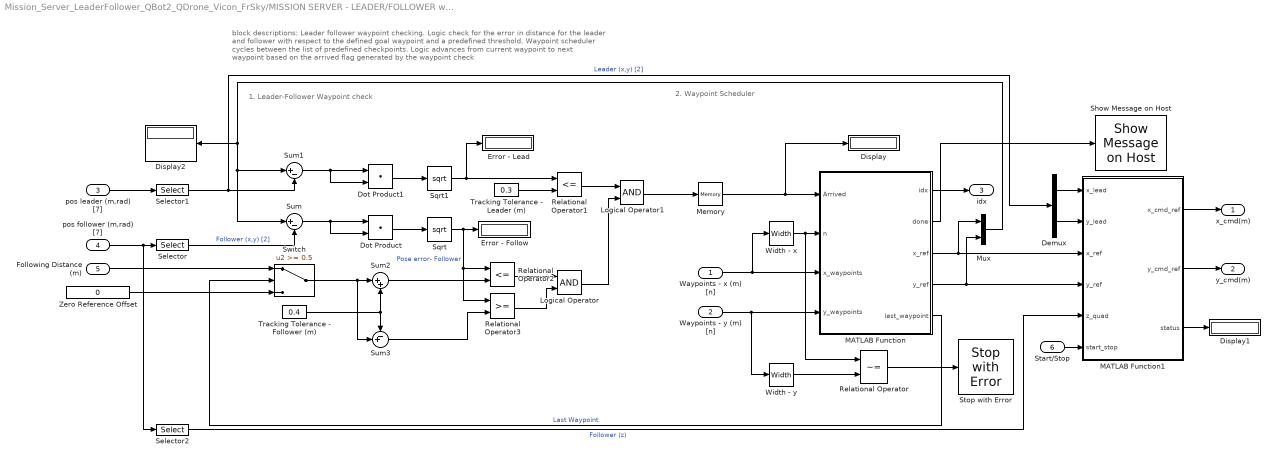
== system Mission_Server_LeaderFollower_QBot2_QDrone_Vicon_FrSky/MISSION SERVER - LEADER/FOLLOWER with QBot 2e and QDrone/Waypoint Scheduler ==
  note: block descriptions:
      | Leader follower waypoint checking. Logic check for the error in distance for the leader and follower with respect to the defined goal waypoint and a predefined threshold.
      | Waypoint scheduler cycles between the list of predefined checkpoints. Logic advances from current waypoint to next waypoint based on the arrived flag generated by the waypoint check
  note: 2. Waypoint Scheduler
  note: 1. Leader-Follower Waypoint check
  Waypoints - x (m) [n] : Inport
  Waypoints - y (m) [n] : Inport  Port=2
  pos leader (m,rad) [7] : Inport  Port=3
  pos follower (m,rad) [7] : Inport  Port=4
  Following Distance (m) : Inport  Port=5
  Start/Stop : Inport  Port=6
  Demux : Demux  Outputs=2
  Display : Display
  Display1 : Display
  Display2 : Display
  Dot Product : DotProduct  InputSameDT=on  OutDataTypeStr=Inherit: Inherit via internal rule
  Dot Product1 : DotProduct  InputSameDT=on  OutDataTypeStr=Inherit: Inherit via internal rule
  Error - Follow : Display
  Error - Lead : Display
  Logical Operator : Logic  AllPortsSameDT=off  OutDataTypeStr=boolean
  Logical Operator1 : Logic  AllPortsSameDT=off  OutDataTypeStr=boolean
  MATLAB Function : MATLAB Function  TreatAsAtomicUnit=on
  MATLAB Function1 : MATLAB Function  TreatAsAtomicUnit=on
  Memory : Memory
  Mux : Mux  Inputs=2
  Relational Operator : RelationalOperator  Operator=~=  OutDataTypeStr=boolean  RndMeth=Nearest
  Relational Operator1 : RelationalOperator  Operator=<=  OutDataTypeStr=boolean  RndMeth=Nearest
  Relational Operator2 : RelationalOperator  Operator=<=  OutDataTypeStr=boolean  RndMeth=Nearest
  Relational Operator3 : RelationalOperator  OutDataTypeStr=boolean  RndMeth=Nearest
  Selector : Selector  InputPortWidth=7  IndexOptions=Index vector (dialog)  Indices=[1 2]  OutputSizes=1
  Selector1 : Selector  InputPortWidth=7  IndexOptions=Index vector (dialog)  Indices=[1 2]  OutputSizes=1
  Selector2 : Selector  InputPortWidth=7  IndexOptions=Index vector (dialog)  Indices=[3]  OutputSizes=1
  Show Message on Host : quarc_library/Sinks/Error Handling/Show Message on Host  message_type=Fixed error message  message_icon=Information  message=Vehicles at final waypoint. Please land QDrone and then stop all models.
      settings: AttributesFormatString="\"%<message>\""  SourceProductName=QUARC Targets
  Sqrt : Sqrt  SaturateOnIntegerOverflow=on
  Sqrt1 : Sqrt  SaturateOnIntegerOverflow=on
  Stop with Error : quarc_library/Sinks/Error Handling/Stop with Error  message_type=Fixed error message  message=Error: Number of x and y waypoints not equal!
      settings: AttributesFormatString="\"%<message>\""  SourceProductName=QUARC Targets
  Sum : Sum  Inputs=|+-
  Sum1 : Sum  Inputs=|+-
  Sum2 : Sum  Inputs=|++
  Sum3 : Sum  Inputs=-+|
  Switch : Switch  Threshold=0.5
  Tracking Tolerance - Follower (m) : Constant  Value=0.4
  Tracking Tolerance - Leader (m) : Constant  Value=0.3
  Width - x : Width
  Width - y : Width
  Zero Reference Offset : Constant  Value=0
  x_cmd(m) : Outport
  y_cmd(m) : Outport  Port=2
  idx : Outport  Port=3
  wires:
  Relational Operator/1 -> Stop with Error/1
  Logical Operator1/1 -> Memory/1
  Memory/1 -> Display/1, MATLAB Function/1(Arrived)
  Width - x/1 -> Relational Operator/1, MATLAB Function/2(n)
  Waypoints - x (m) [n]/1 -> Width - x/1, MATLAB Function/3(x_waypoints)
  Waypoints - y (m) [n]/1 -> Width - y/1, MATLAB Function/4(y_waypoints)
  MATLAB Function/1(idx) -> idx/1
  MATLAB Function/2(done) -> Show Message on Host/1
  MATLAB Function/3(x_ref) -> MATLAB Function1/3(x_ref), Mux/1
  MATLAB Function/4(y_ref) -> MATLAB Function1/4(y_ref), Mux/2
  Width - y/1 -> Relational Operator/2
  Logical Operator/1 -> Logical Operator1/2
  Following Distance (m)/1 -> Switch/1
  MATLAB Function/5(last_waypoint) -> Switch/2  "Last Waypoint"
  Tracking Tolerance - Follower (m)/1 -> Sum3/1, Sum2/2
  Sum2/1 -> Relational Operator2/2
  Zero Reference Offset/1 -> Switch/3
  Relational Operator2/1 -> Logical Operator/1
  Relational Operator3/1 -> Logical Operator/2
  Sum3/1 -> Relational Operator3/2
  Tracking Tolerance - Leader (m)/1 -> Relational Operator1/2
  Sqrt/1 -> Error - Follow/1, Relational Operator2/1, Relational Operator3/1  "Pose error- Follower"
  Relational Operator1/1 -> Logical Operator1/1
  Switch/1 -> Sum2/1, Sum3/2
  pos follower (m,rad) [7]/1 -> Selector2/1, Selector/1
  pos leader (m,rad) [7]/1 -> Selector1/1
  Selector/1 -> Sum/2  "Follower (x,y) [2]"
  Sum/1 -> Dot Product/2, Dot Product/1
  Dot Product/1 -> Sqrt/1
  Sqrt1/1 -> Relational Operator1/1, Error - Lead/1
  Dot Product1/1 -> Sqrt1/1
  Mux/1 -> Sum1/1, Sum/1, Display2/1
  Sum1/1 -> Dot Product1/2, Dot Product1/1
  Selector1/1 -> Demux/1, Sum1/2  "Leader (x,y) [2]"
  Demux/1 -> MATLAB Function1/1(x_lead)
  Demux/2 -> MATLAB Function1/2(y_lead)
  Start/Stop/1 -> MATLAB Function1/6(start_stop)
  MATLAB Function1/1(x_cmd_ref) -> x_cmd(m)/1
  MATLAB Function1/2(y_cmd_ref) -> y_cmd(m)/1
  MATLAB Function1/3(status) -> Display1/1
  Selector2/1 -> MATLAB Function1/5(z_quad)  "Follower (z)"

== system Mission_Server_LeaderFollower_QBot2_QDrone_Vicon_FrSky/MISSION SERVER - LEADER/FOLLOWER with QBot 2e and QDrone/Calculate Home Pose/Enabled Subsystem ==
  "Pose (m, rad ) [4] " : Inport
  Enable : EnablePort
  "Home Pose (m, rad ) [4]" : Outport
  wires:
  "Pose (m, rad ) [4] "/1 -> "Home Pose (m, rad ) [4]"/1

== system Mission_Server_LeaderFollower_QBot2_QDrone_Vicon_FrSky/MISSION SERVER - LEADER/FOLLOWER with QBot 2e and QDrone/Data Server (Localization) /Convention Correction (Vicon Frame to Research Studio Frame) - QBot2e ==
  note: The VICON Global frame and the Research Studio Frame (RSF) are co-located and aligned.
      | The only mapping change is in the re-mapping of the Euler representation from
      | Relateive (Intrinsic) X-Y-Z to Relative Z-Y-X.
  xyz_global (m) [3] : Inport
  rot_global (rad) [3] : Inport  Port=2
  Demux : Demux  Outputs=3
  Euler Angles from Rotation Matrix (Relative ZYX) : quarc_library/Math Operations/Matrices/Euler Angles from Rotation Matrix  menu_order=Relative Z-Y-X
      settings: SourceProductName=QUARC Targets
  Euler Angles to Rotation Matrix (Relative XYZ) : quarc_library/Math Operations/Matrices/Euler Angles to Rotation Matrix  menu_order=Relative X-Y-Z
      settings: SourceProductName=QUARC Targets
  Inverse of Orthonormal Matrix : Math  Operator=transpose  SaturateOnIntegerOverflow=on
  Mux : Mux  Inputs=3
  xyz_RSF (m) [3] : Outport
  rot_RSF (rad) [3] : Outport  Port=2
  R [3x3] : Outport  Port=3
  RT [3x3] : Outport  Port=4
  wires:
  Demux/3 -> Euler Angles to Rotation Matrix (Relative XYZ)/3
  Demux/1 -> Euler Angles to Rotation Matrix (Relative XYZ)/1
  rot_global (rad) [3]/1 -> Demux/1
  Demux/2 -> Euler Angles to Rotation Matrix (Relative XYZ)/2
  xyz_global (m) [3]/1 -> xyz_RSF (m) [3]/1
  Euler Angles from Rotation Matrix (Relative ZYX)/1 -> Mux/3
  Mux/1 -> rot_RSF (rad) [3]/1
  Euler Angles from Rotation Matrix (Relative ZYX)/3 -> Mux/1
  Euler Angles from Rotation Matrix (Relative ZYX)/2 -> Mux/2
  Euler Angles to Rotation Matrix (Relative XYZ)/1 -> Inverse of Orthonormal Matrix/1, R [3x3]/1, Euler Angles from Rotation Matrix (Relative ZYX)/1
  Inverse of Orthonormal Matrix/1 -> RT [3x3]/1

== system Mission_Server_LeaderFollower_QBot2_QDrone_Vicon_FrSky/MISSION SERVER - LEADER/FOLLOWER with QBot 2e and QDrone/Data Server (Localization) /Convention Correction (Vicon Frame to Research Studio Frame) - QDrone ==
  note: The VICON Global frame and the Research Studio Frame (RSF) are co-located and aligned.
      | The only mapping change is in the re-mapping of the Euler representation from
      | Relateive (Intrinsic) X-Y-Z to Relative Z-Y-X.
  xyz_global (m) [3] : Inport
  rot_global (rad) [3] : Inport  Port=2
  Demux : Demux  Outputs=3
  Euler Angles from Rotation Matrix (Relative ZYX) : quarc_library/Math Operations/Matrices/Euler Angles from Rotation Matrix  menu_order=Relative Z-Y-X
      settings: SourceProductName=QUARC Targets
  Euler Angles to Rotation Matrix (Relative XYZ) : quarc_library/Math Operations/Matrices/Euler Angles to Rotation Matrix  menu_order=Relative X-Y-Z
      settings: SourceProductName=QUARC Targets
  Inverse of Orthonormal Matrix : Math  Operator=transpose  SaturateOnIntegerOverflow=on
  Mux : Mux  Inputs=3
  xyz_RSF (m) [3] : Outport
  rot_RSF (rad) [3] : Outport  Port=2
  R [3x3] : Outport  Port=3
  RT [3x3] : Outport  Port=4
  wires:
  Inverse of Orthonormal Matrix/1 -> RT [3x3]/1
  Euler Angles to Rotation Matrix (Relative XYZ)/1 -> Euler Angles from Rotation Matrix (Relative ZYX)/1, R [3x3]/1, Inverse of Orthonormal Matrix/1
  Euler Angles from Rotation Matrix (Relative ZYX)/2 -> Mux/2
  Euler Angles from Rotation Matrix (Relative ZYX)/3 -> Mux/1
  Mux/1 -> rot_RSF (rad) [3]/1
  Euler Angles from Rotation Matrix (Relative ZYX)/1 -> Mux/3
  xyz_global (m) [3]/1 -> xyz_RSF (m) [3]/1
  Demux/2 -> Euler Angles to Rotation Matrix (Relative XYZ)/2
  rot_global (rad) [3]/1 -> Demux/1
  Demux/1 -> Euler Angles to Rotation Matrix (Relative XYZ)/1
  Demux/3 -> Euler Angles to Rotation Matrix (Relative XYZ)/3

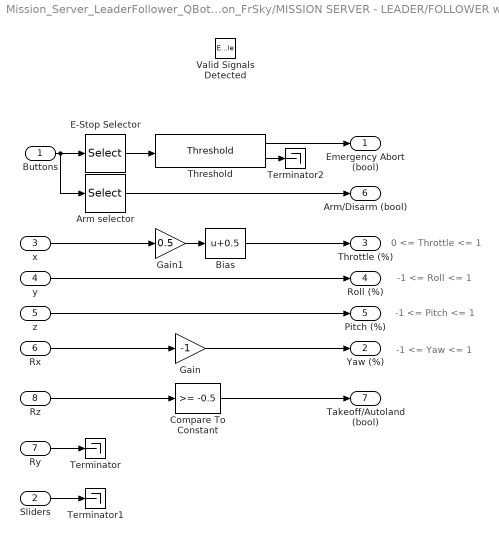
== system Mission_Server_LeaderFollower_QBot2_QDrone_Vicon_FrSky/MISSION SERVER - LEADER/FOLLOWER with QBot 2e and QDrone/JOYSTICK/FrSKYMapping ==
  note: -1 <= Pitch <= 1
  note: -1 <= Roll <= 1
  note: 0 <= Throttle <= 1
  note: -1 <= Yaw <= 1
  Buttons : Inport
  Sliders : Inport  Port=2
  x : Inport  Port=3
  y : Inport  Port=4
  z : Inport  Port=5
  Rx : Inport  Port=6
  Ry : Inport  Port=7
  Rz : Inport  Port=8
  Valid Signals Detected : EnablePort
  Arm selector : Selector  InputPortWidth=32  IndexOptions=Index vector (dialog)  Indices=[2]  OutputSizes=1
  Bias : Bias  Bias=0.5
  Compare To Constant : simulink/Logic and Bit Operations/Compare To Constant  relop=>=  const=-0.5  OutDataTypeStr=boolean
  E-Stop Selector : Selector  InputPortWidth=32  IndexOptions=Index vector (dialog)  Indices=[1]  OutputSizes=1
  Gain : Gain  Gain=-1
  Gain1 : Gain  Gain=0.5
  Terminator : Terminator
  Terminator1 : Terminator
  Terminator2 : Terminator
  Threshold : quarc_library/Discontinuities/Threshold  operator=>=  param_src=Specify via dialog  threshold=0.5  duration=0.2
      settings: SourceProductName=QUARC Targets
  Emergency Abort (bool) : Outport
  Yaw (%) : Outport  Port=2
  Throttle (%) : Outport  Port=3
  Roll (%) : Outport  Port=4
  Pitch (%) : Outport  Port=5
  "Arm/Disarm (bool) " : Outport  Port=6
  Takeoff/Autoland (bool) : Outport  Port=7
  wires:
  Bias/1 -> Throttle (%)/1
  Gain1/1 -> Bias/1
  Gain/1 -> Yaw (%)/1
  Threshold/2 -> Terminator2/1
  Threshold/1 -> Emergency Abort (bool)/1
  Compare To Constant/1 -> Takeoff/Autoland (bool)/1
  Rz/1 -> Compare To Constant/1
  E-Stop Selector/1 -> Threshold/1
  Sliders/1 -> Terminator1/1
  Ry/1 -> Terminator/1
  Rx/1 -> Gain/1
  z/1 -> Pitch (%)/1
  y/1 -> Roll (%)/1
  x/1 -> Gain1/1
  Arm selector/1 -> "Arm/Disarm (bool) "/1
  Buttons/1 -> E-Stop Selector/1, Arm selector/1
